simulink model "DSF_A3"  (R2022b)
settings: configuration reference "CommonModelConfiguration" (kept outside this file)
undefined symbols (not defined in the file or in its folder): AccSts1, AdjSpdLimnMsg1, AdjSpdLimnSts2, AdjSpdLimnWarnCoding, AsyLaneChgPsbl1, AsyLaneChgSts2, AsyLaneChgTyp2, AvlStsForAsyLaneChg, AvlStsForLatAutDrv5, AvlStsForLongAutDrv4, AvlStsForSteerSpprt1, Boolean, CarModSts1, CllsnAidPostEve3, CrsCtrlrMsg1, CrsCtrlrSts1, CrvtSpdAdj2, CtryForRoadSgn1, DrvrSpprtFct, E_CommonStatus, E_DSF_Event, E_DSF_Messages, E_DSF_Value, FctSts2, FctStsSpdCtrl, HmiAutnmsSts1, LaneDetnSts1, LCFG_SetSpeedMinKPH, LCFG_SetSpeedMinKPH_A3, LvlWarn1, MplLvlVisWarn1, NoYesCrit1, OffOnNotAvlSrvRqrd, OnOff1, PsdNotPsd, SetSpdSelnForAutDrv1, SpdAdjmtEveForAutDrv, SpdUnit1, SteerIntvSts1, SteerStsForAutDrv3, SteerWarnReqForAutDrv1, SteerWarnSts1, UndrtknPrevnWarnReq, UsgModSts1, VehDetd1, VehSpdIndcdUnit, VisWarnReq1
libraries: simulink x127
(part 3 of 3)

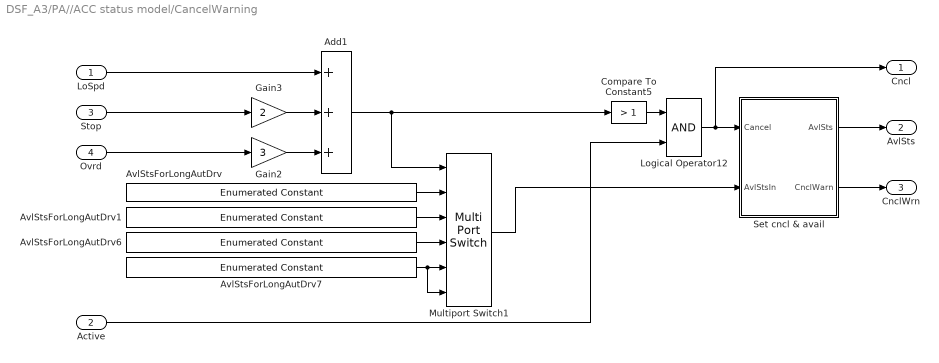
== system DSF_A3/PA//ACC status model/CancelWarning ==
  LoSpd : Inport
  Active : Inport  Port=2
  Stop : Inport  Port=3
  Ovrd : Inport  Port=4
  Add1 : Sum  Inputs=+++
  AvlStsForLongAutDrv : simulink/Sources/Enumerated Constant  OutDataTypeStr=Enum: AvlStsForLongAutDrv4  Value=AvlStsForLongAutDrv4.AvlStsForLongAutDrv4_NoMsg  SampleTime=inf
  AvlStsForLongAutDrv1 : simulink/Sources/Enumerated Constant  OutDataTypeStr=Enum: AvlStsForLongAutDrv4  Value=AvlStsForLongAutDrv4.AvlStsForLongAutDrv4_NoVehAhd  SampleTime=inf
  AvlStsForLongAutDrv6 : simulink/Sources/Enumerated Constant  OutDataTypeStr=Enum: AvlStsForLongAutDrv4  Value=AvlStsForLongAutDrv4.AvlStsForLongAutDrv4_HldTiMaxExcdd  SampleTime=inf
  AvlStsForLongAutDrv7 : simulink/Sources/Enumerated Constant  OutDataTypeStr=Enum: AvlStsForLongAutDrv4  Value=AvlStsForLongAutDrv4.AvlStsForLongAutDrv4_OvrdTiMaxExcdd  SampleTime=inf
  Compare To Constant5 : simulink/Logic and Bit Operations/Compare To Constant  relop=>  const=1  OutDataTypeStr=boolean
  Gain2 : Gain  Gain=3  OutDataTypeStr=double
  Gain3 : Gain  Gain=2  OutDataTypeStr=double
  Logical Operator12 : Logic  AllPortsSameDT=off  OutDataTypeStr=boolean
  Multiport Switch1 : MultiPortSwitch  DataPortOrder=Zero-based contiguous  Inputs=5  DiagnosticForDefault=None  zeroidx=on  SaturateOnIntegerOverflow=off  InputSameDT=off
  Set cncl & avail : Stateflow chart  TreatAsAtomicUnit=on
  Cncl : Outport
  AvlSts : Outport  Port=2
  CnclWrn : Outport  Port=3
  wires:
  Active/1 -> Logical Operator12/2
  Logical Operator12/1 -> Cncl/1, Set cncl & avail/1(Cancel)
  Gain3/1 -> Add1/2
  Gain2/1 -> Add1/3
  LoSpd/1 -> Add1/1
  Ovrd/1 -> Gain2/1
  Stop/1 -> Gain3/1
  Set cncl & avail/1(AvlSts) -> AvlSts/1
  Set cncl & avail/2(CnclWarn) -> CnclWrn/1
  Add1/1 -> Multiport Switch1/1, Compare To Constant5/1
  AvlStsForLongAutDrv7/1 -> Multiport Switch1/6, Multiport Switch1/5
  AvlStsForLongAutDrv6/1 -> Multiport Switch1/4
  AvlStsForLongAutDrv1/1 -> Multiport Switch1/3
  AvlStsForLongAutDrv/1 -> Multiport Switch1/2
  Multiport Switch1/1 -> Set cncl & avail/2(AvlStsIn)
  Compare To Constant5/1 -> Logical Operator12/1

== stateflow chart DSF_A3/ISA model/Chart1 ==
  state WARNING_ON
    en, du: SET_SpdLimAudWarnReq = OnOff1.OnOff1_On;
  state WARNING_OFF
    en, du: SET_SpdLimAudWarnReq = OnOff1.OnOff1_Off;
  (default) -> WARNING_OFF
  WARNING_OFF -> WARNING_ON : %Speed limit exceeded
      | [hasChangedTo(SpdLimitExcd, true)]
  WARNING_ON -> WARNING_OFF : %Speed limit no longer exceeded or request times out
      | [hasChangedTo(SpdLimitExcd, false) || after(2, sec)]
  data: SpdLimitExcd input; SET_SpdLimAudWarnReq output

== stateflow chart DSF_A3/Speed limit//SLA model/SLA//SpdLim ==
  state NEW_SPEED_LIMIT
    entry:
    SET_SetSpdSelnForAutDrv =...
    SetSpdSelnForAutDrv1.SetSpdSelnForAutDrv1_KeepSetSpdValPrsnt;
    SET_SpdLimAdpvActv = OnOff1.OnOff1_Off;
  state SHOW
  state ACTIVATE_SLA
    entry:
    SET_SpdLimAdpvActv = OnOff1.OnOff1_On;
  (default) -> NEW_SPEED_LIMIT : {SET_SpdLimFirst = SpdLimFirst;
      | SET_SpdLimSec = SpdLimSec;}
  (junction 94) -> SHOW [order 2]
  NEW_SPEED_LIMIT -> (junction 94) [order 2] : [PushUp==PsdNotPsd.PsdNotPsd_Psd &&...
      | SET_SpdLimFirst <= 150]
      | {SET_SpdLimSec =...
      |  SET_SpdLimFirst + 10;}
  (junction 94) -> SHOW [order 1] : [SET_SpdLimSec==150]
      | {SET_SpdLimSec = 254;}
  SHOW -> ACTIVATE_SLA : [after(2, sec)]
      | {SET_SpdLimFirst = SET_SpdLimSec;
      | SET_SpdLimSec = 0; SET_SetSpdSelnForAutDrv =...
      | SetSpdSelnForAutDrv1.SetSpdSelnForAutDrv1_AdjSetSpdToSpdLimPrsnt;}
  (junction 91) -> SHOW [order 1] : [SL_Sts==AdjSpdLimnSts2.AdjSpdLimnSts2_Actv]
  (junction 97) -> (junction 91) [order 2]
  NEW_SPEED_LIMIT -> (junction 97) [order 1] : [PushDown==PsdNotPsd.PsdNotPsd_Psd &&...
      | SET_SpdLimFirst >= 20]...
      | {SET_SpdLimSec =...
      | SET_SpdLimFirst - 10;}
  (junction 97) -> (junction 91) [order 1] : [SET_SpdLimSec>130]
      | {SET_SpdLimSec = 130;}
  (junction 91) -> ACTIVATE_SLA [order 2] : {SET_SetSpdSelnForAutDrv =...
      | SetSpdSelnForAutDrv1.SetSpdSelnForAutDrv1_AdjSetSpdToCmngSpdLim;}
  NEW_SPEED_LIMIT -> ACTIVATE_SLA [order 3] : [(hasChangedTo(AccSts, AccSts1.AccSts1_Actv) || hasChangedTo(CC_Sts, CrsCtrlrSts1.CrsCtrlrSts1_Actv) ||...
      | hasChangedTo(SL_Sts, AdjSpdLimnSts2.AdjSpdLimnSts2_Actv)) && SetSpeed<SpdLimFirst]
      | {SET_SetSpdSelnForAutDrv = SetSpdSelnForAutDrv1.SetSpdSelnForAutDrv1_AdjSetSpdToSpdLimPrsnt;}
  (junction 83) -> NEW_SPEED_LIMIT [order 1] : [SET_SpdLimSec~=0]
      | {SET_SpdLimFirst = SET_SpdLimSec;
      | SET_SpdLimSec = 0;}
  ACTIVATE_SLA -> (junction 83) : [after(3, sec)]
  (junction 83) -> NEW_SPEED_LIMIT [order 2]
  data: SET_SpdLimSec output; SET_SpdLimFirst output; PushUp input; PushDown input; SpdLimFirst input; SpdLimSec input; SET_SetSpdSelnForAutDrv output; SET_SpdLimAdpvActv output; AccSts input; CC_Sts input; SL_Sts input; SetSpeed input

== stateflow chart DSF_A3/ISA model/Chart ==
  state ISA_OFF
    en, du: SET_SpdLimAudWarnSts = WarnSts.WarnSts_OFF;
  state ISA_ON
    en, du: SET_SpdLimAudWarnSts = WarnSts.WarnSts_ON;
  (default) -> ISA_ON
  ISA_ON -> ISA_OFF : %Button L2 pressed
      | [INT_SWSInputData_Button == E_SWSButton.BtnL2Req &&...
      | hasChangedTo(INT_SWSInputData_Event, E_SWSEvent.Push)]
  ISA_OFF -> ISA_ON : %Button L2 pressed
      | [INT_SWSInputData_Button == E_SWSButton.BtnL2Req &&...
      | hasChangedTo(INT_SWSInputData_Event, E_SWSEvent.Push)]
  data: INT_SWSInputData_Button input; INT_SWSInputData_Event input; SET_SpdLimAudWarnSts output

== stateflow chart DSF_A3/LCA model/LaneChgLe ==
  state TURNING_OFF
    en, du:
    TurnPeriod = false;
    Cancel = false;
  state TURNING_ON
    en, du:
    TurnPeriod = true;
  state TURNING_CANCEL
    en, du:
    TurnPeriod = false;
    Cancel = true;
  (default) -> TURNING_OFF
  TURNING_OFF -> TURNING_ON : %Indicator on
      | [hasChangedTo(TurnSignal, 1) && Psbl]
  TURNING_ON -> TURNING_OFF [order 1] : %Lane changed cancelled or finished
      | [hasChangedTo(Cncl, 1) || after(15, sec)]
  TURNING_CANCEL -> TURNING_OFF : [after(3, sec)]
  TURNING_ON -> TURNING_CANCEL [order 2] : %Cancelled by driver, indicator off
      | [hasChangedTo(TurnSignal, 0)]
  data: TurnSignal input; TurnPeriod output; Cncl input; Psbl input; Cancel output

== stateflow chart DSF_A3/LCA model/LaneChgRi ==
  state TURNING_OFF
    en, du:
    TurnPeriod = false;
    Cancel = false;
  state TURNING_ON
    en, du:
    TurnPeriod = true;
  state TURNING_CANCEL
    en, du:
    TurnPeriod = false;
    Cancel = true;
  (default) -> TURNING_OFF
  TURNING_OFF -> TURNING_ON : %Indicator on
      | [hasChangedTo(TurnSignal, 1) && Psbl]
  TURNING_ON -> TURNING_OFF [order 1] : %Lane changed cancelled or finished
      | [hasChangedTo(Cncl, 1) || after(15, sec)]
  TURNING_CANCEL -> TURNING_OFF : [after(3, sec)]
  TURNING_ON -> TURNING_CANCEL [order 2] : %Cancelled by driver, indicator off
      | [hasChangedTo(TurnSignal, 0)]
  data: TurnSignal input; TurnPeriod output; Cncl input; Psbl input; Cancel output

== stateflow chart DSF_A3/PA//ACC status model/Override timeout ==
  state TIMER_ON
  state TIMER_OFF
    en, du: Timeout = false;
  state TIMEOUT
    en, du: Timeout = true;
  (default) -> TIMER_OFF
  TIMER_OFF -> TIMER_ON : %Timer on
      | [hasChangedTo(Set, true)]
  TIMER_ON -> TIMER_OFF [order 2] : %Timer off
      | [hasChangedTo(Set, false)]
  TIMER_ON -> TIMEOUT [order 1] : %Timeout reached
      | [after(Time, sec)]
  TIMEOUT -> TIMER_OFF : %Reset timer
      | [after(1, sec)]
  data: Set input; Timeout output; Time input

== stateflow chart DSF_A3/PA//ACC status model/Stop timeout ==
  state TIMEOUT_OFF
    en, du: Timeout = false;
  state TIMER_ON
  state TIMEOUT_ON
    en, du: Timeout = true;
  (default) -> TIMEOUT_OFF
  TIMEOUT_OFF -> TIMER_ON : %Stop mode initiated
      | [hasChangedTo(State, AccSts1.AccSts1_Stop)]
  TIMER_ON -> TIMEOUT_OFF [order 1] : %Activated, reset
      | [hasChangedTo(State, AccSts1.AccSts1_Actv)]
  TIMER_ON -> TIMEOUT_ON [order 2] : %Timeout reached
      | [after(Time, sec)]
  TIMEOUT_ON -> TIMEOUT_OFF : %Reset timer
      | [after(1, sec)]
  data: State input; Timeout output; Time input

== stateflow chart DSF_A3/HOW model/Level1 timer ==
  state TIMER_ON
  state TIMER_OFF
    en, du: Timeout = false;
  state TIMEOUT
    en, du: Timeout = true;
  (default) -> TIMER_OFF
  TIMER_OFF -> TIMER_ON : %Timer on
      | [hasChangedTo(Set, true)]
  TIMER_ON -> TIMER_OFF [order 2] : %Timer off
      | [hasChangedTo(Set, false)]
  TIMEOUT -> TIMER_OFF : %Reset timer
      | [hasChangedTo(Set, false)]
  TIMER_ON -> TIMEOUT [order 1] : %Timeout reached
      | [after(Time, sec)]
  data: Set input; Timeout output; Time input

== stateflow chart DSF_A3/HOW model/Level2 timer ==
  state TIMER_ON
  state TIMER_OFF
    en, du: Timeout = false;
  state TIMEOUT
    en, du: Timeout = true;
  (default) -> TIMER_OFF
  TIMER_OFF -> TIMER_ON : %Timer on
      | [hasChangedTo(Set, true)]
  TIMER_ON -> TIMER_OFF [order 2] : %Timer off
      | [hasChangedTo(Set, false)]
  TIMEOUT -> TIMER_OFF : %Reset timer
      | [hasChangedTo(Set, false)]
  TIMER_ON -> TIMEOUT [order 1] : %Timeout reached
      | [after(Time, sec)]
  data: Set input; Timeout output; Time input

== stateflow chart DSF_A3/HOW model/ESA//deactivate timer ==
  state TIMER_ON
  state TIMER_OFF
    en, du: Timeout = false;
  state TIMEOUT
    en, du: Timeout = true;
  (default) -> TIMER_OFF
  TIMER_OFF -> TIMER_ON : %Timer on
      | [hasChangedTo(Set, true)]
  TIMER_ON -> TIMER_OFF [order 2] : %Timer off
      | [hasChangedTo(Set, false)]
  TIMER_ON -> TIMEOUT [order 1] : %Timeout reached
      | [after(Time, sec)]
  (junction 19) -> TIMER_OFF : [after(3, sec)]
  TIMEOUT -> (junction 19) : %Reset timer
      | [hasChangedTo(Set, false) ||...
      | hasChangedTo(PA_act, false)]
  data: Set input; Timeout output; Time input; PA_act input

== stateflow chart DSF_A3/CC model/CC_State ==
  state CC_OFF
    en, du: State = CrsCtrlrSts1.CrsCtrlrSts1_Off;
  state CC_ACTIVE
    en, du: State = CrsCtrlrSts1.CrsCtrlrSts1_Actv;
  state CC_STBY
    en, du: State = CrsCtrlrSts1.CrsCtrlrSts1_Stb;
  (default) -> CC_OFF
  CC_OFF -> CC_STBY : %CC selected
      | [CrsCtrlFctSeld==...
      | DrvrCrsCtrlFctSeldTyp.DrvrCrsCtrlFctSeldTyp_CrsCtrlFct]
  CC_STBY -> CC_OFF [order 2] : %CC not selected
      | [CrsCtrlFctSeld~=...
      | DrvrCrsCtrlFctSeldTyp.DrvrCrsCtrlFctSeldTyp_CrsCtrlFct]
  CC_STBY -> CC_ACTIVE [order 1] : %Activate CC
      | [hasChangedTo(Activate, true)]
  CC_ACTIVE -> CC_STBY : %CC standby
      | [hasChangedTo(Deactivate, true)]
  data: CrsCtrlFctSeld input; Activate input; State output; Deactivate input

== stateflow chart DSF_A3/PA//ACC status model/ACC_State ==
  state ACC_OFF
    en, du: State = AccSts1.AccSts1_Off;
  state ACC_ACTIVE
    en, du: State = AccSts1.AccSts1_Actv;
  state ACC_STBY
    en, du: State = AccSts1.AccSts1_Stb;
  state STOPPED
  state ACC_STOP
    en, du: State = AccSts1.AccSts1_Stop;
  (default) -> ACC_OFF
  ACC_OFF -> ACC_STBY : %ACC selected
      | [CrsCtrlFctSeld==...
      | DrvrCrsCtrlFctSeldTyp.DrvrCrsCtrlFctSeldTyp_AccFct]
  ACC_STBY -> ACC_OFF [order 2] : %ACC not selected
      | [CrsCtrlFctSeld~=...
      | DrvrCrsCtrlFctSeldTyp.DrvrCrsCtrlFctSeldTyp_AccFct]
  ACC_STBY -> ACC_ACTIVE [order 1] : %Activate ACC
      | [hasChangedTo(Activate, true)]
  ACC_ACTIVE -> ACC_STBY [order 2] : %ACC standby
      | [hasChangedTo(Deactivate, true)]
  ACC_STOP -> ACC_STBY [order 2] : %Stop mode timeout
      | [hasChangedTo(Deactivate, true)]
  ACC_ACTIVE -> STOPPED [order 1] : [TgtSpd==0]
  STOPPED -> ACC_ACTIVE [order 2] : [TgtSpd~=0]
  ACC_STOP -> ACC_ACTIVE [order 1] : [hasChangedTo(Activate, true)]
  STOPPED -> ACC_STOP [order 1] : [after(3, sec)]
  data: TgtSpd input; CrsCtrlFctSeld input; Activate input; State output; Deactivate input

== stateflow chart DSF_A3/SL model/SL_State ==
  state SL_OFF
    en, du: State = AdjSpdLimnSts2.AdjSpdLimnSts2_Off;
  state SL_ACTIVE
    en, du: State = AdjSpdLimnSts2.AdjSpdLimnSts2_Actv;
  state SL_STANDBY
    en, du: State = AdjSpdLimnSts2.AdjSpdLimnSts2_Stb;
  state SL_OVERRIDDEN
    en, du: State = AdjSpdLimnSts2.AdjSpdLimnSts2_Ovrd;
  (default) -> SL_OFF
  SL_OFF -> SL_STANDBY : %SL selected
      | [CrsCtrlFctSeld==...
      | DrvrCrsCtrlFctSeldTyp.DrvrCrsCtrlFctSeldTyp_SpdLimFct]
  SL_STANDBY -> SL_OFF [order 2] : %SL not selected
      | [CrsCtrlFctSeld~=...
      | DrvrCrsCtrlFctSeldTyp.DrvrCrsCtrlFctSeldTyp_SpdLimFct]
  SL_STANDBY -> SL_ACTIVE [order 1] : %Activate SL
      | [hasChangedTo(Activate, true)]
  SL_ACTIVE -> SL_STANDBY [order 1] : %SL standby
      | [hasChangedTo(Deactivate, true)]
  SL_OVERRIDDEN -> SL_STANDBY [order 2] : [hasChangedTo(Deactivate, true)]
  SL_ACTIVE -> SL_OVERRIDDEN [order 2] : [CrsCtrlOvrdn==...
      | OnOff1.OnOff1_On]
  SL_OVERRIDDEN -> SL_ACTIVE [order 1] : [CrsCtrlOvrdn==...
      | OnOff1.OnOff1_Off]
  data: CrsCtrlFctSeld input; Activate input; State output; Deactivate input; CrsCtrlOvrdn input

== stateflow chart DSF_A3/PA//ACC status model/Misuse ==
  state STEER_OFF
    en, du: NoSteer = true;
  state STEER_ON
    en, du: NoSteer = false;
  (default) -> STEER_ON
  STEER_ON -> STEER_OFF : %Hands off wheel for too long
      | [hasChangedTo(EmgStop, true)]
  data: EmgStop input; NoSteer output

== stateflow chart DSF_A3/PA//ACC status model/CancelWarning/Set cncl & avail ==
  state HOLD_AVAILABILITY
    entry:
    CnclWarn = NoYesCrit1.NoYesCrit1_Yes;
    AvlSts = AvlStsIn;
  state CURRENT_AVAILABILITY
    en, du:
    CnclWarn = NoYesCrit1.NoYesCrit1_No;
    AvlSts = AvlStsIn;
  (default) -> CURRENT_AVAILABILITY
  CURRENT_AVAILABILITY -> HOLD_AVAILABILITY : %Cancel condition
      | [hasChangedTo(Cancel, true)]
  HOLD_AVAILABILITY -> CURRENT_AVAILABILITY : %Hold timeout
      | [after(2, sec)]
  data: AvlSts output; Cancel input; CnclWarn output; AvlStsIn input

== stateflow chart DSF_A3/PA//ACC status model/PA_State ==
  state PA_STBY
    en, du: State = OnOff1.OnOff1_Off;
  state PA_ACTIVE
    en, du: State = OnOff1.OnOff1_Off;
  state STEER_ASSIST_ACTIVE
    en, du: State = OnOff1.OnOff1_On;
  (default) -> PA_STBY
  PA_STBY -> PA_ACTIVE : %Activate steer assist
      | [hasChangedTo(Activate, true)]
  PA_ACTIVE -> PA_STBY [order 2] : %Deactivate steer assist
      | [hasChangedTo(Deactivate, true)]
  STEER_ASSIST_ACTIVE -> PA_STBY [order 2] : %Deactivate steer assist
      | [hasChangedTo(Deactivate, true)]
  PA_ACTIVE -> STEER_ASSIST_ACTIVE [order 1] : % Activate steering if available
      | [Unavailable==false]
  STEER_ASSIST_ACTIVE -> PA_ACTIVE [order 1] : % Deactivate steering if unavailable
      | [Unavailable==true]
  data: Activate input; State output; Deactivate input; Unavailable input
